simulink model "settaDemo"  (R2020a)
settings: Solver=VariableStepAuto  StartTime=0.0  StopTime=0.1  RelTol=1e-3
settings Model: Creator=bzhan  LastModifiedBy=bzhan

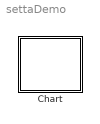
== system settaDemo ==
  Chart : Stateflow chart  TreatAsAtomicUnit=on

== stateflow chart settaDemo/Chart ==
  settings: updateMethod=DISCRETE  sampleTime=0.1
  state A [parallel]
    en: x=1;
    settings: executionOrder=1
    (junction 3) -> A : /{send(E,B)}
    A -> A [order 2] : {fprintf("C\n");}
    A -> (junction 3) [order 1] : [x==1]/{fprintf("B\n");}
  state B [parallel]
    du: fprintf("D\n");
    settings: executionOrder=2
    B -> B : E{fprintf("A\n");}
  data: x local
  events: E local FUNCTION_CALL_EVENT
